simulink model "cyclo_converter"  (R2013b)
settings: Solver=ode45  StartTime=0.0  StopTime=0.1  RelTol=1e-3
undefined symbols (not defined in the file): alpha
libraries: powerlib x15, powerlib_meascontrol x1
settings Model: Creator=SAI KUMAR  LastModifiedBy=SAI KUMAR

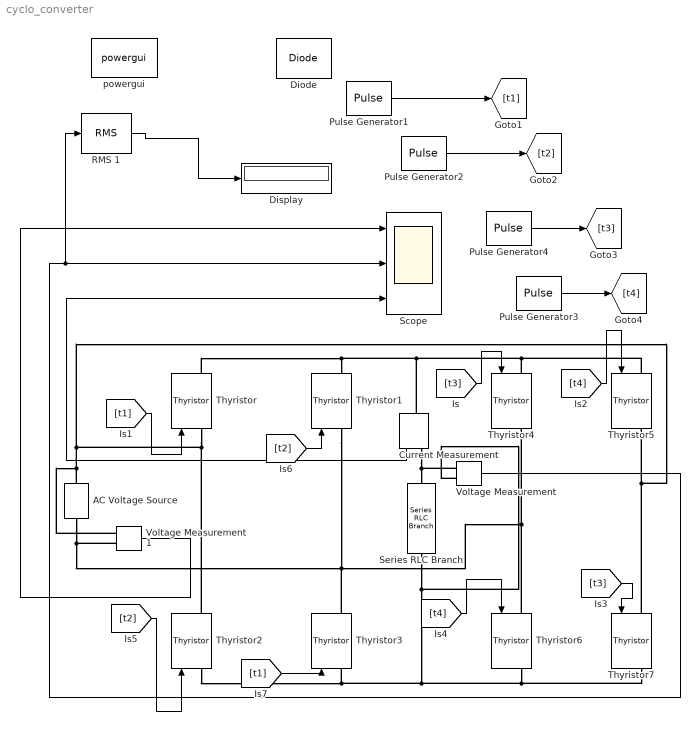
== system cyclo_converter ==
  AC Voltage Source : powerlib/Electrical Sources/AC Voltage Source  Amplitude=220*sqrt(2)  Phase=0  Frequency=50  SampleTime=0  Measurements=None
  Current Measurement : powerlib/Measurements/Current Measurement  PhasorSimulation=off  OutputType=Complex  PSBequivalent=0
  Diode : powerlib/Power Electronics/Diode  Ron=0.001  Lon=0  Vf=0.8  IC=0  UseSnubber=off  Rs=500  Cs=250e-9  Measurements=on
  Display : Display
  Pulse Generator1 : DiscretePulseGenerator  PulseType=Time based  Amplitude=5  Period=0.06  PhaseDelay=((0.02/360)*alpha)
  Pulse Generator2 : DiscretePulseGenerator  PulseType=Time based  Amplitude=5  Period=0.06  PhaseDelay=0.01+((0.02/360)*alpha)
  Pulse Generator3 : DiscretePulseGenerator  PulseType=Time based  Amplitude=5  Period=0.06  PhaseDelay=0.04+((0.02/360)*alpha)
  Pulse Generator4 : DiscretePulseGenerator  PulseType=Time based  Amplitude=5  Period=0.06  PulseWidth=10  PhaseDelay=0.05+((0.02/360)*alpha)
  RMS 1 : powerlib_meascontrol/Measurements/RMS  TrueRMS=on  Freq=16.66667  RMSInit=0  Ts=0
  Scope : Scope  NumInputPorts=3
      settings: YMin=-5~-5~-5  YMax=5~5~5
  Series RLC Branch : powerlib/Elements/Series RLC Branch  LConnTagsString=__new0  RConnTagsString=__new0  BranchType=RL  Resistance=10  Inductance=10e-3  SetiL0=off  InitialCurrent=0  Capacitance=1e-6  Setx0=off  InitialVoltage=0  Measurements=None
  Thyristor{,1..7} (8 alike) : powerlib/Power Electronics/Thyristor  Ron=0.001  Lon=0  Vf=0.8  IC=0  Rs=500  Cs=250e-9  Measurements=on
  Voltage Measurement : powerlib/Measurements/Voltage Measurement  PhasorSimulation=off  OutputType=Complex  PSBequivalent=0
  Voltage Measurement1 : powerlib/Measurements/Voltage Measurement  PhasorSimulation=off  OutputType=Complex  PSBequivalent=0
  powergui : powerlib/powergui  Priority=1  SimulationMode=Continuous  SolverType=Tustin  SampleTime=50e-6  frequency=60  SPID=off  DisableSnubberDevices=off  DisableRonSwitches=off  DisableVfSwitches=off  SwTol=0  Interpol=off  DisplayEquations=off  frequencyindice=50  Pbase=100e6  ErrMax=1e-4  Iterations=50  UnitsV=kV  UnitsW=MW  FunctionMessages=off  echomessages=off  HookPort=off  EnableUseOfTLC=off  x0status=blocks  RestoreLinks=warning  ResistiveCurrentMeasurement=off  Frange=[0:2:500]  Ylog=off  Xlog=on  ShowGrid=off  save=off  variable=ZData  ZoomFFT=off  StartTime=0.0  cycles=1  DisplayStyle=1  fundamental=60  FreqAxis=off  MaxFrequency=1000  frequencyindicesteady=1  RmsSteady=1  display=off  Ts=0  methode=off
  wires:
  Voltage Measurement/1 -> RMS 1/1, Scope/2
  Pulse Generator1/1 -> [t1]
  Pulse Generator2/1 -> [t2]
  Current Measurement/1 -> Scope/3
  Voltage Measurement1/1 -> Scope/1
  [t4] -> Thyristor6/1
  [t3] -> Thyristor7/1
  [t4] -> Thyristor5/1
  [t3] -> Thyristor4/1
  [t1] -> Thyristor/1
  [t2] -> Thyristor2/1
  [t1] -> Thyristor3/1
  [t2] -> Thyristor1/1
  Pulse Generator4/1 -> [t3]
  Pulse Generator3/1 -> [t4]
  RMS 1/1 -> Display/1
  connections:
  Thyristor2/LConn1 -- Voltage Measurement/LConn2 -- Series RLC Branch/RConn1 -- Thyristor7/RConn1 -- Thyristor6/RConn1 -- Thyristor3/LConn1
  Thyristor/RConn1 -- Current Measurement/LConn1 -- Thyristor5/LConn1 -- Thyristor4/LConn1 -- Thyristor1/RConn1
  Thyristor6/LConn1 -- Voltage Measurement1/LConn2 -- AC Voltage Source/LConn1 -- Thyristor1/LConn1 -- Thyristor3/RConn1 -- Thyristor4/RConn1
  Thyristor7/LConn1 -- Voltage Measurement1/LConn1 -- AC Voltage Source/RConn1 -- Thyristor/LConn1 -- Thyristor2/RConn1 -- Thyristor5/RConn1
  Current Measurement/RConn1 -- Voltage Measurement/LConn1 -- Series RLC Branch/LConn1
